simulink model "Prova_inversione_Linearized"  (R2015a)
settings: Solver=ode45  StartTime=0.0  StopTime=10.0  RelTol=1e-3
values from neighbouring files (symbols this model uses):
  b = 0.55/2    (= 0.275)    [TiltCopter_Parameters.m]
  degtorad = pi/180    (= 0.0174532925199)    [TiltCopter_Parameters.m]
  Kq = Cq*ro*A*R^3    (= 2.88925724261e-07)    [TiltCopter_Parameters.m]
  Kt = Ct*ro*A*R^2    (= 2.46191978476e-05)    [TiltCopter_Parameters.m]
  m_servo = p(1)    [TiltCopter_Parameters.m]
  omega_hover = OMEhov    [TiltCopter_Parameters.m]
  q_servo = p(2)    [TiltCopter_Parameters.m]
  x1 = [m q]    [TiltCopter_Parameters.m]
settings Model: Creator=Claudio  LastModifiedBy=Claudio

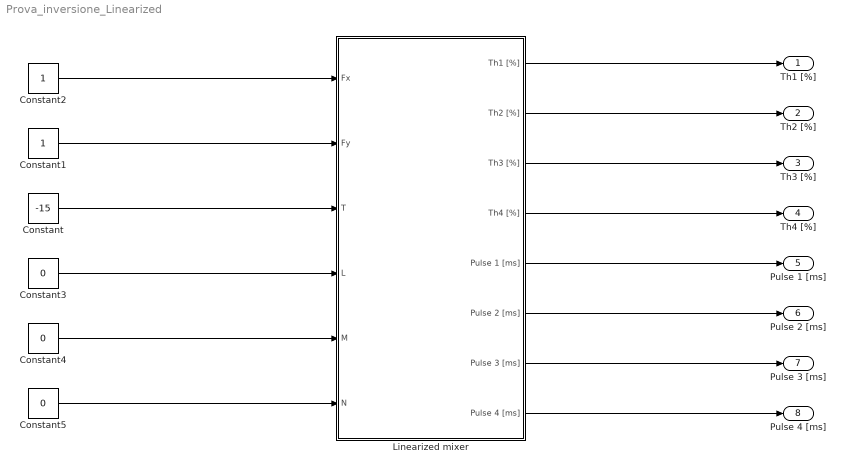
== system Prova_inversione_Linearized ==
  Constant : Constant  Value=-15
  Constant1 : Constant
  Constant2 : Constant
  Constant3 : Constant  Value=0
  Constant4 : Constant  Value=0
  Constant5 : Constant  Value=0
  Linearized mixer : Subsystem
  Th1 [%] : Outport
  Th2 [%] : Outport  Port=2
  Th3 [%] : Outport  Port=3
  Th4 [%] : Outport  Port=4
  Pulse 1 [ms] : Outport  Port=5
  Pulse 2 [ms] : Outport  Port=6
  Pulse 3 [ms] : Outport  Port=7
  Pulse 4 [ms] : Outport  Port=8
  wires:
  Constant2/1 -> Linearized mixer/1(Fx)
  Constant1/1 -> Linearized mixer/2(Fy)
  Constant/1 -> Linearized mixer/3(T)
  Constant3/1 -> Linearized mixer/4(L)
  Constant4/1 -> Linearized mixer/5(M)
  Constant5/1 -> Linearized mixer/6(N)
  Linearized mixer/1(Th1 [%]) -> Th1 [%]/1
  Linearized mixer/2(Th2 [%]) -> Th2 [%]/1
  Linearized mixer/3(Th3 [%]) -> Th3 [%]/1
  Linearized mixer/4(Th4 [%]) -> Th4 [%]/1
  Linearized mixer/5(Pulse 1 [ms]) -> Pulse 1 [ms]/1
  Linearized mixer/6(Pulse 2 [ms]) -> Pulse 2 [ms]/1
  Linearized mixer/7(Pulse 3 [ms]) -> Pulse 3 [ms]/1
  Linearized mixer/8(Pulse 4 [ms]) -> Pulse 4 [ms]/1

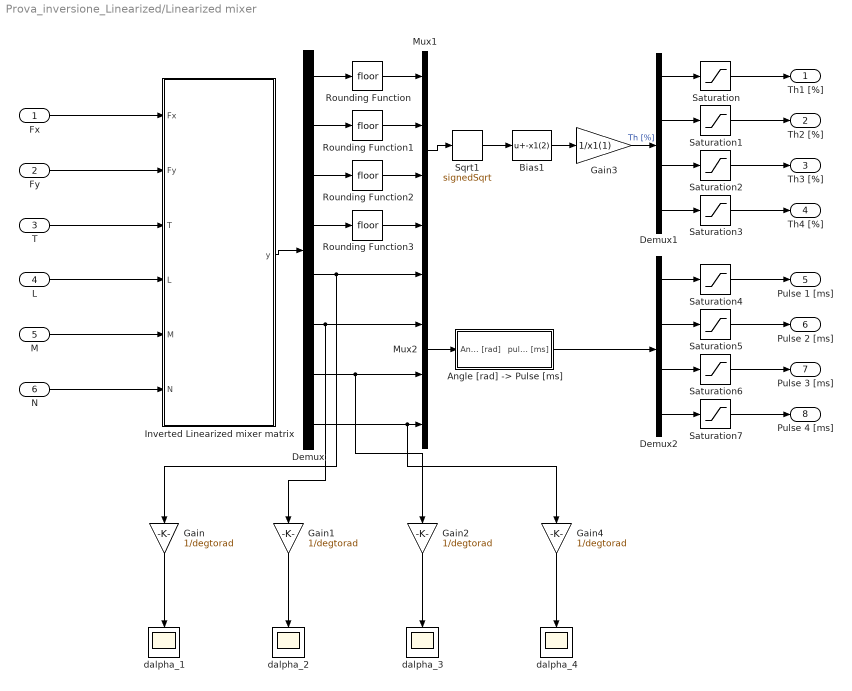
== system Prova_inversione_Linearized/Linearized mixer ==
  Fx : Inport
  Fy : Inport  Port=2
  T : Inport  Port=3
  L : Inport  Port=4
  M : Inport  Port=5
  N : Inport  Port=6
  "Angle [rad] -> Pulse [ms]" : Subsystem
  Bias1 : Bias  Bias=-x1(2)
  Demux : Demux  Outputs=8
  Demux1 : Demux
  Demux2 : Demux
  Gain{,1..2,4} (4 alike) : Gain  Gain=1/degtorad
  Gain3 : Gain  Gain=1/x1(1)
  Inverted Linearized mixer matrix : MATLAB Function  TreatAsAtomicUnit=on
  Mux1 : Mux
  Mux2 : Mux
  Rounding Function{,1..3} (4 alike) : Rounding
  Saturation{,1..3} (4 alike) : Saturate  UpperLimit=100  LowerLimit=0
  Saturation{4..7} (4 alike) : Saturate  UpperLimit=2000  LowerLimit=1000
  Sqrt1 : Sqrt  Operator=signedSqrt  SaturateOnIntegerOverflow=on
  dalpha_{1..4} (4 alike) : Scope
      dalpha_3 settings: SaveName=ScopeData6
      dalpha_4 settings: SaveName=ScopeData7
  Th1 [%] : Outport
  Th2 [%] : Outport  Port=2
  Th3 [%] : Outport  Port=3
  Th4 [%] : Outport  Port=4
  Pulse 1 [ms] : Outport  Port=5
  Pulse 2 [ms] : Outport  Port=6
  Pulse 3 [ms] : Outport  Port=7
  Pulse 4 [ms] : Outport  Port=8
  wires:
  Rounding Function/1 -> Mux1/1
  Saturation6/1 -> Pulse 3 [ms]/1
  Fx/1 -> Inverted Linearized mixer matrix/1(Fx)
  L/1 -> Inverted Linearized mixer matrix/4(L)
  Inverted Linearized mixer matrix/1(y) -> Demux/1
  Fy/1 -> Inverted Linearized mixer matrix/2(Fy)
  N/1 -> Inverted Linearized mixer matrix/6(N)
  T/1 -> Inverted Linearized mixer matrix/3(T)
  M/1 -> Inverted Linearized mixer matrix/5(M)
  Demux2/1 -> Saturation4/1
  Demux2/3 -> Saturation6/1
  Demux/4 -> Rounding Function3/1
  Demux/2 -> Rounding Function1/1
  Saturation2/1 -> Th3 [%]/1
  Demux1/2 -> Saturation1/1
  Demux1/1 -> Saturation/1
  Demux1/3 -> Saturation2/1
  Demux1/4 -> Saturation3/1
  Saturation1/1 -> Th2 [%]/1
  Gain3/1 -> Demux1/1  "Th [%]"
  Sqrt1/1 -> Bias1/1
  Mux1/1 -> Sqrt1/1
  Demux/1 -> Rounding Function/1
  Bias1/1 -> Gain3/1
  Saturation3/1 -> Th4 [%]/1
  Saturation/1 -> Th1 [%]/1
  Demux2/2 -> Saturation5/1
  Rounding Function1/1 -> Mux1/2
  Rounding Function3/1 -> Mux1/4
  Demux/7 -> Gain2/1, Mux2/3
  Demux/5 -> Gain/1, Mux2/1
  Demux/6 -> Mux2/2, Gain1/1
  Mux2/1 -> "Angle [rad] -> Pulse [ms]"/1(Angle [rad])
  Demux2/4 -> Saturation7/1
  Demux/3 -> Rounding Function2/1
  Demux/8 -> Gain4/1, Mux2/4
  "Angle [rad] -> Pulse [ms]"/1(pulse [ms]) -> Demux2/1
  Saturation4/1 -> Pulse 1 [ms]/1
  Saturation5/1 -> Pulse 2 [ms]/1
  Saturation7/1 -> Pulse 4 [ms]/1
  Gain1/1 -> dalpha_2/1
  Gain/1 -> dalpha_1/1
  Gain2/1 -> dalpha_3/1
  Gain4/1 -> dalpha_4/1
  Rounding Function2/1 -> Mux1/3

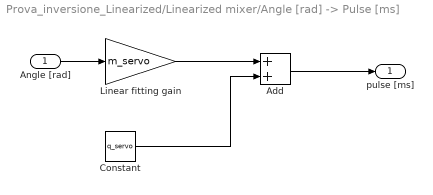
== system Prova_inversione_Linearized/Linearized mixer/Angle [rad] -> Pulse [ms] ==
  Angle [rad] : Inport
  Add : Sum
  Constant : Constant  Value=q_servo
  Linear fitting gain : Gain  Gain=m_servo
  pulse [ms] : Outport
  wires:
  Angle [rad]/1 -> Linear fitting gain/1
  Constant/1 -> Add/2
  Linear fitting gain/1 -> Add/1
  Add/1 -> pulse [ms]/1

== matlab function Prova_inversione_Linearized/Linearized mixer/Inverted Linearized mixer matrix ==
  data: Fx input; Fy input; T input; L input; M input; N input; y output; omega_hover parameter; Kt parameter; Kq parameter; b parameter
function y = fcn(Fx,Fy,T,L,M,N,omega_hover,Kt,Kq,b)
%#codegen

omega_hover_sq = omega_hover^2;

% Linearized Mixer matrix (equilibrium points: omega = omega hover, alpha =
% 0

MM_param_jaco =[    0,     0,     0,    0,                   0,  -Kt*omega_hover_sq,                   0,   Kt*omega_hover_sq;
    0,     0,     0,    0,   Kt*omega_hover_sq,                   0,  -Kt*omega_hover_sq,                   0;
  -Kt,   -Kt,   -Kt,  -Kt,                   0,                   0,                   0,                   0;
    0, -Kt*b,     0, Kt*b,                   0,  -Kq*omega_hover_sq,                   0,   Kq*omega_hover_sq;
 Kt*b,     0, -Kt*b,    0,  -Kq*omega_hover_sq,                   0,   Kq*omega_hover_sq,                   0;
   Kq,   -Kq,    Kq,  -Kq, Kt*b*omega_hover_sq, Kt*b*omega_hover_sq, Kt*b*omega_hover_sq, Kt*b*omega_hover_sq];

% Compute the column vector result
result = pinv(MM_param_jaco)*[Fx;Fy;T;L;M;N];
y = result;
